simulink subsystem "nonlinear_model_2"  (R2026a)
settings: Solver=VariableStepAuto
undefined symbols (not defined in the file): b, d, m, P
settings Model: Creator=Kiril  LastModifiedBy=User

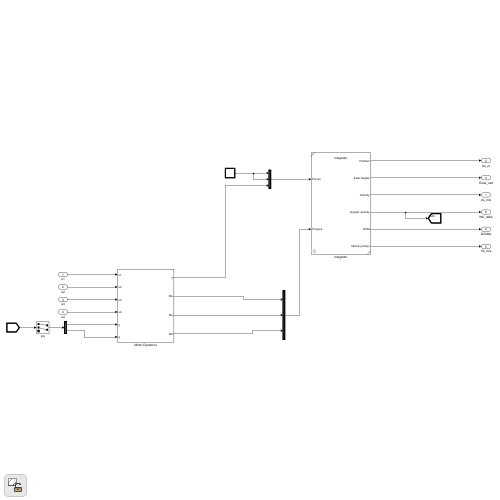
[thumbnail: Simulink's stored preview of the top-level diagram]
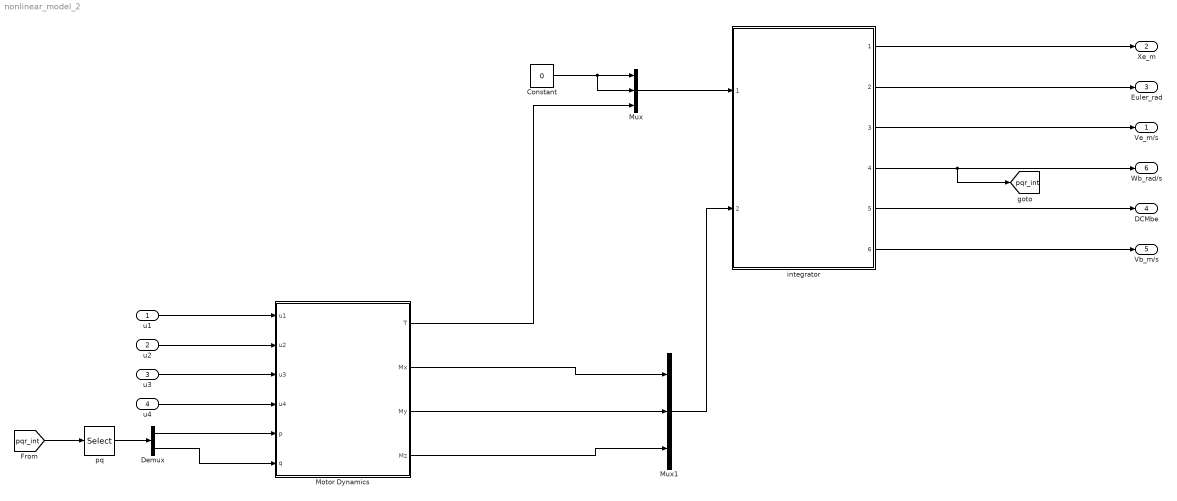
== system nonlinear_model_2 ==
  u1 : Inport
  u2 : Inport  Port=2
  u3 : Inport  Port=3
  u4 : Inport  Port=4
  Constant : Constant  Value=0
  Demux : Demux  Outputs=2
  Motor Dynamics : Subsystem
  Mux : Mux  Inputs=3
  Mux1 : Mux  Inputs=3
  integrator : Subsystem  ReferencedSubsystem=integrator  Mass=m  Inertia=P.I  Pos=Sim.Initial_Position  Velocity=Sim.Initial_Velocity_Body  Orient=Sim.Initial_Euler_Angles_Rad  AngVelocity=Sim.Initial_Body_Angular_Rates_Rads
  pq : Selector  InputPortWidth=3  IndexOptions=Index vector (dialog)  Indices=[1 2]  OutputSizes=1
  Ve_m/s : Outport
  Xe_m : Outport  Port=2
  Euler_rad : Outport  Port=3
  DCMbe : Outport  Port=4
  Vb_m/s : Outport  Port=5
  Wb_rad/s : Outport  Port=6
  tag scope: pqr_int=global
  wires:
  u1/1 -> Motor Dynamics/1(u1)
  u2/1 -> Motor Dynamics/2(u2)
  u3/1 -> Motor Dynamics/3(u3)
  u4/1 -> Motor Dynamics/4(u4)
  [pqr_int] -> pq/1
  pq/1 -> Demux/1
  Demux/1 -> Motor Dynamics/5(p)
  Demux/2 -> Motor Dynamics/6(q)
  integrator/5 -> DCMbe/1
  Motor Dynamics/1(T) -> Mux/3
  Motor Dynamics/2(Mx) -> Mux1/1
  Motor Dynamics/3(My) -> Mux1/2
  Motor Dynamics/4(Mz) -> Mux1/3
  Mux1/1 -> integrator/2
  integrator/3 -> Ve_m/s/1
  integrator/1 -> Xe_m/1
  integrator/2 -> Euler_rad/1
  integrator/6 -> Vb_m/s/1
  integrator/4 -> [pqr_int], Wb_rad/s/1
  Mux/1 -> integrator/1
  Constant/1 -> Mux/1, Mux/2

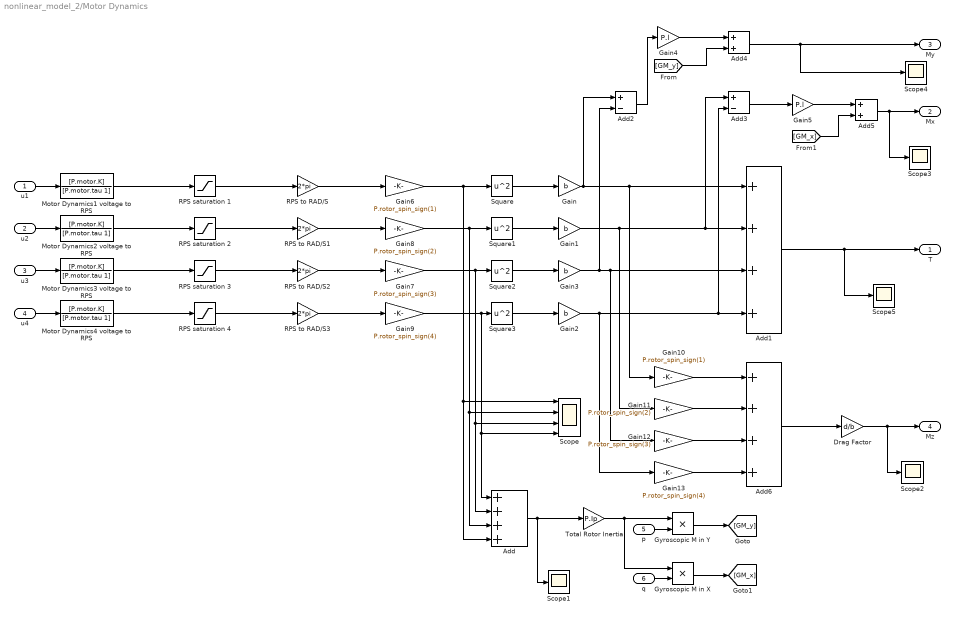
== system nonlinear_model_2/Motor Dynamics ==
  u1 : Inport
  u2 : Inport  Port=2
  u3 : Inport  Port=3
  u4 : Inport  Port=4
  p : Inport  Port=5
  q : Inport  Port=6
  Add : Sum  Inputs=++++
  Add1 : Sum  Inputs=++++
  Add2 : Sum  Inputs=+-
  Add3 : Sum  Inputs=+-
  Add4 : Sum
  Add5 : Sum
  Add6 : Sum  Inputs=++++
  Drag Factor : Gain  Gain=d/b
  Gain{,1..3} (4 alike) : Gain  Gain=b
  Gain10 : Gain  Gain=P.rotor_spin_sign(1)
  Gain11 : Gain  Gain=P.rotor_spin_sign(2)
  Gain12 : Gain  Gain=P.rotor_spin_sign(3)
  Gain13 : Gain  Gain=P.rotor_spin_sign(4)
  Gain4 : Gain  Gain=P.l
  Gain5 : Gain  Gain=P.l
  Gain6 : Gain  Gain=P.rotor_spin_sign(1)
  Gain7 : Gain  Gain=P.rotor_spin_sign(3)
  Gain8 : Gain  Gain=P.rotor_spin_sign(2)
  Gain9 : Gain  Gain=P.rotor_spin_sign(4)
  Gyroscopic M in X : Product
  Gyroscopic M in Y : Product
  Motor Dynamics1 voltage to RPS : TransferFcn  Numerator=[P.motor.K]  Denominator=[P.motor.tau 1]
  Motor Dynamics2 voltage to RPS : TransferFcn  Numerator=[P.motor.K]  Denominator=[P.motor.tau 1]
  Motor Dynamics3 voltage to RPS : TransferFcn  Numerator=[P.motor.K]  Denominator=[P.motor.tau 1]
  Motor Dynamics4 voltage to RPS : TransferFcn  Numerator=[P.motor.K]  Denominator=[P.motor.tau 1]
  RPS saturation {1..4} (4 alike) : Saturate  UpperLimit=P.motor.rps_max  LowerLimit=P.motor.rps_min
  RPS to RAD/S{,1..3} (4 alike) : Gain  Gain=2*pi
  Scope : Scope  NumInputPorts=4
      settings: ActiveDisplayYMinimum=-93.322674018396327  ActiveDisplayYMaximum=105.52486202765351  DataLoggingVariableName=ScopeData3
  Scope{1..5} (5 alike) : Scope
      Scope1 settings: ActiveDisplayYMinimum=-1  ActiveDisplayYMaximum=1  DataLoggingVariableName=ScopeData5
      Scope2 settings: ActiveDisplayYMinimum=-1  ActiveDisplayYMaximum=1  DataLoggingVariableName=ScopeData4
      Scope3 settings: ActiveDisplayYMinimum=-1  ActiveDisplayYMaximum=1  DataLoggingVariableName=ScopeData6
      Scope4 settings: ActiveDisplayYMinimum=-1  ActiveDisplayYMaximum=1  DataLoggingVariableName=ScopeData7
      Scope5 settings: ActiveDisplayYMinimum=-0.00014611451482860572  ActiveDisplayYMaximum=0.0013150306334574517  DataLoggingVariableName=ScopeData8
  Square{,1..3} (4 alike) : Math  Operator=square
  Total Rotor Inertia : Gain  Gain=P.Ip
  T : Outport
  Mx : Outport  Port=2
  My : Outport  Port=3
  Mz : Outport  Port=4
  wires:
  u1/1 -> Motor Dynamics1 voltage to RPS/1
  u2/1 -> Motor Dynamics2 voltage to RPS/1
  u3/1 -> Motor Dynamics3 voltage to RPS/1
  u4/1 -> Motor Dynamics4 voltage to RPS/1
  Add/1 -> Total Rotor Inertia/1, Scope1/1
  p/1 -> Gyroscopic M in Y/2
  Total Rotor Inertia/1 -> Gyroscopic M in X/1, Gyroscopic M in Y/1
  q/1 -> Gyroscopic M in X/2
  Square/1 -> Gain/1
  Square1/1 -> Gain1/1
  Square2/1 -> Gain3/1
  Square3/1 -> Gain2/1
  Add1/1 -> T/1, Scope5/1
  Add2/1 -> Gain4/1
  Gain4/1 -> Add4/1
  [GM_y] -> Add4/2
  Add3/1 -> Gain5/1
  Gain5/1 -> Add5/1
  [GM_x] -> Add5/2
  Add6/1 -> Drag Factor/1
  Add5/1 -> Mx/1, Scope3/1
  Add4/1 -> My/1, Scope4/1
  Drag Factor/1 -> Mz/1, Scope2/1
  Gain6/1 -> Add/4, Scope/1, Square/1
  Gain7/1 -> Square2/1, Add/2, Scope/3
  Gain8/1 -> Add/3, Scope/2, Square1/1
  Gain9/1 -> Add/1, Scope/4, Square3/1
  Gain/1 -> Add2/1, Gain10/1, Add1/1
  Gain1/1 -> Gain11/1, Add3/1, Add1/2
  Gain3/1 -> Add2/2, Gain12/1, Add1/3
  Gain2/1 -> Gain13/1, Add3/2, Add1/4
  Gain10/1 -> Add6/1
  Gain11/1 -> Add6/2
  Gain12/1 -> Add6/3
  Gain13/1 -> Add6/4
  RPS to RAD/S/1 -> Gain6/1
  RPS to RAD/S1/1 -> Gain8/1
  RPS to RAD/S2/1 -> Gain7/1
  RPS to RAD/S3/1 -> Gain9/1
  RPS saturation 4/1 -> RPS to RAD/S3/1
  Motor Dynamics4 voltage to RPS/1 -> RPS saturation 4/1
  RPS saturation 3/1 -> RPS to RAD/S2/1
  Motor Dynamics3 voltage to RPS/1 -> RPS saturation 3/1
  RPS saturation 2/1 -> RPS to RAD/S1/1
  Motor Dynamics2 voltage to RPS/1 -> RPS saturation 2/1
  RPS saturation 1/1 -> RPS to RAD/S/1
  Motor Dynamics1 voltage to RPS/1 -> RPS saturation 1/1
  Gyroscopic M in X/1 -> [GM_x]
  Gyroscopic M in Y/1 -> [GM_y]
